simulink model "dedisp_sync"  (R2013b)
settings: Solver=FixedStepDiscrete  SolverMode=SingleTasking  StartTime=0.0  StopTime=10.0  RelTol=1e-3
undefined symbols (not defined in the file): pfb_coeff_gen_calc
libraries: xbsIndex_r4 x14646, casper_library_misc x70, casper_library_delays x55, dspsigops x16, xps_library x2, casper_library_pfbs x2
(part 19 of 146)

== system dedisp_sync/Parallel_Dedispersor_v11/Dedispersor_v2_1 ==
  Data : Inport
  Valid : Inport  Port=2
  Counter : xbsIndex_r4/Counter  cnt_type=Free Running  cnt_to=Inf  operation=Up  start_count=0  cnt_by_val=1  arith_type=Unsigned  n_bits=4  bin_pt=0  load_pin=off  rst=off  en=on  explicit_period=on  period=1  dbl_ovrd=off  use_behavioral_HDL=off  implementation=Fabric  block_type=counter
  Mux : xbsIndex_r4/Mux  inputs=16  en=off  latency=0  precision=Full  arith_type=Unsigned  n_bits=16  bin_pt=14  quantization=Truncate  overflow=Wrap  dbl_ovrd=off  block_type=mux
  detector_block_v2 : Subsystem  AncestorBlock=honestlibrary/detector_block_v2  mask(Basic block for FRB detection){chn=0, lat=1, nbits=4, behavioral=on}
      mask prompts: chn "Channel"; lat "Latency"; nbits "Number of Bits (Counter)"; behavioral "behavioral delay"
      mask help:
      | Delays a certain channel a number of latency clock cycles, according to the fixed DM table.
      | This version incorporates an internal counter (nbits) to know when store or give a certain value.
      mask init:
      | detector_block_init_v2(gcb,'chn',chn,'lat',lat,'nbits',nbits,'behavioral', behavioral)
      settings: AttributesFormatString=Channel: 0, Delay: 1
  detector_block_v21 : Subsystem  AncestorBlock=honestlibrary/detector_block_v2  mask(Basic block for FRB detection){chn=1, lat=2, nbits=4, behavioral=on}
      mask prompts: chn "Channel"; lat "Latency"; nbits "Number of Bits (Counter)"; behavioral "behavioral delay"
      mask help:
      | Delays a certain channel a number of latency clock cycles, according to the fixed DM table.
      | This version incorporates an internal counter (nbits) to know when store or give a certain value.
      mask init:
      | detector_block_init_v2(gcb,'chn',chn,'lat',lat,'nbits',nbits,'behavioral', behavioral)
      settings: AttributesFormatString=Channel: 1, Delay: 2
  detector_block_v210 : Subsystem  AncestorBlock=honestlibrary/detector_block_v2  mask(Basic block for FRB detection){chn=10, lat=11, nbits=4, behavioral=on}
      mask prompts: chn "Channel"; lat "Latency"; nbits "Number of Bits (Counter)"; behavioral "behavioral delay"
      mask help:
      | Delays a certain channel a number of latency clock cycles, according to the fixed DM table.
      | This version incorporates an internal counter (nbits) to know when store or give a certain value.
      mask init:
      | detector_block_init_v2(gcb,'chn',chn,'lat',lat,'nbits',nbits,'behavioral', behavioral)
      settings: AttributesFormatString=Channel: 10, Delay: 11
  detector_block_v211 : Subsystem  AncestorBlock=honestlibrary/detector_block_v2  mask(Basic block for FRB detection){chn=11, lat=12, nbits=4, behavioral=on}
      mask prompts: chn "Channel"; lat "Latency"; nbits "Number of Bits (Counter)"; behavioral "behavioral delay"
      mask help:
      | Delays a certain channel a number of latency clock cycles, according to the fixed DM table.
      | This version incorporates an internal counter (nbits) to know when store or give a certain value.
      mask init:
      | detector_block_init_v2(gcb,'chn',chn,'lat',lat,'nbits',nbits,'behavioral', behavioral)
      settings: AttributesFormatString=Channel: 11, Delay: 12
  detector_block_v212 : Subsystem  AncestorBlock=honestlibrary/detector_block_v2  mask(Basic block for FRB detection){chn=12, lat=13, nbits=4, behavioral=on}
      mask prompts: chn "Channel"; lat "Latency"; nbits "Number of Bits (Counter)"; behavioral "behavioral delay"
      mask help:
      | Delays a certain channel a number of latency clock cycles, according to the fixed DM table.
      | This version incorporates an internal counter (nbits) to know when store or give a certain value.
      mask init:
      | detector_block_init_v2(gcb,'chn',chn,'lat',lat,'nbits',nbits,'behavioral', behavioral)
      settings: AttributesFormatString=Channel: 12, Delay: 13
  detector_block_v213 : Subsystem  AncestorBlock=honestlibrary/detector_block_v2  mask(Basic block for FRB detection){chn=13, lat=14, nbits=4, behavioral=on}
      mask prompts: chn "Channel"; lat "Latency"; nbits "Number of Bits (Counter)"; behavioral "behavioral delay"
      mask help:
      | Delays a certain channel a number of latency clock cycles, according to the fixed DM table.
      | This version incorporates an internal counter (nbits) to know when store or give a certain value.
      mask init:
      | detector_block_init_v2(gcb,'chn',chn,'lat',lat,'nbits',nbits,'behavioral', behavioral)
      settings: AttributesFormatString=Channel: 13, Delay: 14
  detector_block_v214 : Subsystem  AncestorBlock=honestlibrary/detector_block_v2  mask(Basic block for FRB detection){chn=14, lat=15, nbits=4, behavioral=on}
      mask prompts: chn "Channel"; lat "Latency"; nbits "Number of Bits (Counter)"; behavioral "behavioral delay"
      mask help:
      | Delays a certain channel a number of latency clock cycles, according to the fixed DM table.
      | This version incorporates an internal counter (nbits) to know when store or give a certain value.
      mask init:
      | detector_block_init_v2(gcb,'chn',chn,'lat',lat,'nbits',nbits,'behavioral', behavioral)
      settings: AttributesFormatString=Channel: 14, Delay: 15
  detector_block_v215 : Subsystem  AncestorBlock=honestlibrary/detector_block_v2  mask(Basic block for FRB detection){chn=15, lat=16, nbits=4, behavioral=on}
      mask prompts: chn "Channel"; lat "Latency"; nbits "Number of Bits (Counter)"; behavioral "behavioral delay"
      mask help:
      | Delays a certain channel a number of latency clock cycles, according to the fixed DM table.
      | This version incorporates an internal counter (nbits) to know when store or give a certain value.
      mask init:
      | detector_block_init_v2(gcb,'chn',chn,'lat',lat,'nbits',nbits,'behavioral', behavioral)
      settings: AttributesFormatString=Channel: 15, Delay: 16
  detector_block_v22 : Subsystem  AncestorBlock=honestlibrary/detector_block_v2  mask(Basic block for FRB detection){chn=2, lat=3, nbits=4, behavioral=on}
      mask prompts: chn "Channel"; lat "Latency"; nbits "Number of Bits (Counter)"; behavioral "behavioral delay"
      mask help:
      | Delays a certain channel a number of latency clock cycles, according to the fixed DM table.
      | This version incorporates an internal counter (nbits) to know when store or give a certain value.
      mask init:
      | detector_block_init_v2(gcb,'chn',chn,'lat',lat,'nbits',nbits,'behavioral', behavioral)
      settings: AttributesFormatString=Channel: 2, Delay: 3
  detector_block_v23 : Subsystem  AncestorBlock=honestlibrary/detector_block_v2  mask(Basic block for FRB detection){chn=3, lat=4, nbits=4, behavioral=on}
      mask prompts: chn "Channel"; lat "Latency"; nbits "Number of Bits (Counter)"; behavioral "behavioral delay"
      mask help:
      | Delays a certain channel a number of latency clock cycles, according to the fixed DM table.
      | This version incorporates an internal counter (nbits) to know when store or give a certain value.
      mask init:
      | detector_block_init_v2(gcb,'chn',chn,'lat',lat,'nbits',nbits,'behavioral', behavioral)
      settings: AttributesFormatString=Channel: 3, Delay: 4
  detector_block_v24 : Subsystem  AncestorBlock=honestlibrary/detector_block_v2  mask(Basic block for FRB detection){chn=4, lat=5, nbits=4, behavioral=on}
      mask prompts: chn "Channel"; lat "Latency"; nbits "Number of Bits (Counter)"; behavioral "behavioral delay"
      mask help:
      | Delays a certain channel a number of latency clock cycles, according to the fixed DM table.
      | This version incorporates an internal counter (nbits) to know when store or give a certain value.
      mask init:
      | detector_block_init_v2(gcb,'chn',chn,'lat',lat,'nbits',nbits,'behavioral', behavioral)
      settings: AttributesFormatString=Channel: 4, Delay: 5
  detector_block_v25 : Subsystem  AncestorBlock=honestlibrary/detector_block_v2  mask(Basic block for FRB detection){chn=5, lat=6, nbits=4, behavioral=on}
      mask prompts: chn "Channel"; lat "Latency"; nbits "Number of Bits (Counter)"; behavioral "behavioral delay"
      mask help:
      | Delays a certain channel a number of latency clock cycles, according to the fixed DM table.
      | This version incorporates an internal counter (nbits) to know when store or give a certain value.
      mask init:
      | detector_block_init_v2(gcb,'chn',chn,'lat',lat,'nbits',nbits,'behavioral', behavioral)
      settings: AttributesFormatString=Channel: 5, Delay: 6
  detector_block_v26 : Subsystem  AncestorBlock=honestlibrary/detector_block_v2  mask(Basic block for FRB detection){chn=6, lat=7, nbits=4, behavioral=on}
      mask prompts: chn "Channel"; lat "Latency"; nbits "Number of Bits (Counter)"; behavioral "behavioral delay"
      mask help:
      | Delays a certain channel a number of latency clock cycles, according to the fixed DM table.
      | This version incorporates an internal counter (nbits) to know when store or give a certain value.
      mask init:
      | detector_block_init_v2(gcb,'chn',chn,'lat',lat,'nbits',nbits,'behavioral', behavioral)
      settings: AttributesFormatString=Channel: 6, Delay: 7
  detector_block_v27 : Subsystem  AncestorBlock=honestlibrary/detector_block_v2  mask(Basic block for FRB detection){chn=7, lat=8, nbits=4, behavioral=on}
      mask prompts: chn "Channel"; lat "Latency"; nbits "Number of Bits (Counter)"; behavioral "behavioral delay"
      mask help:
      | Delays a certain channel a number of latency clock cycles, according to the fixed DM table.
      | This version incorporates an internal counter (nbits) to know when store or give a certain value.
      mask init:
      | detector_block_init_v2(gcb,'chn',chn,'lat',lat,'nbits',nbits,'behavioral', behavioral)
      settings: AttributesFormatString=Channel: 7, Delay: 8
  detector_block_v28 : Subsystem  AncestorBlock=honestlibrary/detector_block_v2  mask(Basic block for FRB detection){chn=8, lat=9, nbits=4, behavioral=on}
      mask prompts: chn "Channel"; lat "Latency"; nbits "Number of Bits (Counter)"; behavioral "behavioral delay"
      mask help:
      | Delays a certain channel a number of latency clock cycles, according to the fixed DM table.
      | This version incorporates an internal counter (nbits) to know when store or give a certain value.
      mask init:
      | detector_block_init_v2(gcb,'chn',chn,'lat',lat,'nbits',nbits,'behavioral', behavioral)
      settings: AttributesFormatString=Channel: 8, Delay: 9
  detector_block_v29 : Subsystem  AncestorBlock=honestlibrary/detector_block_v2  mask(Basic block for FRB detection){chn=9, lat=10, nbits=4, behavioral=on}
      mask prompts: chn "Channel"; lat "Latency"; nbits "Number of Bits (Counter)"; behavioral "behavioral delay"
      mask help:
      | Delays a certain channel a number of latency clock cycles, according to the fixed DM table.
      | This version incorporates an internal counter (nbits) to know when store or give a certain value.
      mask init:
      | detector_block_init_v2(gcb,'chn',chn,'lat',lat,'nbits',nbits,'behavioral', behavioral)
      settings: AttributesFormatString=Channel: 9, Delay: 10
  Output : Outport
  wires:
  Mux/1 -> Output/1
  detector_block_v215/1(Out1) -> Mux/17
  detector_block_v214/1(Out1) -> Mux/16
  detector_block_v213/1(Out1) -> Mux/15
  detector_block_v212/1(Out1) -> Mux/14
  detector_block_v211/1(Out1) -> Mux/13
  detector_block_v210/1(Out1) -> Mux/12
  detector_block_v29/1(Out1) -> Mux/11
  detector_block_v28/1(Out1) -> Mux/10
  detector_block_v27/1(Out1) -> Mux/9
  detector_block_v26/1(Out1) -> Mux/8
  detector_block_v25/1(Out1) -> Mux/7
  detector_block_v24/1(Out1) -> Mux/6
  detector_block_v23/1(Out1) -> Mux/5
  detector_block_v22/1(Out1) -> Mux/4
  detector_block_v21/1(Out1) -> Mux/3
  detector_block_v2/1(Out1) -> Mux/2
  Counter/1 -> Mux/1
  Valid/1 -> Counter/1, detector_block_v215/2(Valid), detector_block_v214/2(Valid), detector_block_v213/2(Valid), detector_block_v212/2(Valid), detector_block_v211/2(Valid), detector_block_v210/2(Valid), detector_block_v29/2(Valid), detector_block_v28/2(Valid), detector_block_v27/2(Valid), detector_block_v26/2(Valid), detector_block_v25/2(Valid), detector_block_v24/2(Valid), detector_block_v23/2(Valid), detector_block_v22/2(Valid), detector_block_v21/2(Valid), detector_block_v2/2(Valid)
  Data/1 -> detector_block_v215/1(Data), detector_block_v214/1(Data), detector_block_v213/1(Data), detector_block_v212/1(Data), detector_block_v211/1(Data), detector_block_v210/1(Data), detector_block_v29/1(Data), detector_block_v28/1(Data), detector_block_v27/1(Data), detector_block_v26/1(Data), detector_block_v25/1(Data), detector_block_v24/1(Data), detector_block_v23/1(Data), detector_block_v22/1(Data), detector_block_v21/1(Data), detector_block_v2/1(Data)

== system dedisp_sync/Parallel_Dedispersor_v11/Dedispersor_v2_2 ==
  Data : Inport
  Valid : Inport  Port=2
  Counter : xbsIndex_r4/Counter  cnt_type=Free Running  cnt_to=Inf  operation=Up  start_count=0  cnt_by_val=1  arith_type=Unsigned  n_bits=4  bin_pt=0  load_pin=off  rst=off  en=on  explicit_period=on  period=1  dbl_ovrd=off  use_behavioral_HDL=off  implementation=Fabric  block_type=counter
  Mux : xbsIndex_r4/Mux  inputs=16  en=off  latency=0  precision=Full  arith_type=Unsigned  n_bits=16  bin_pt=14  quantization=Truncate  overflow=Wrap  dbl_ovrd=off  block_type=mux
  detector_block_v2 : Subsystem  AncestorBlock=honestlibrary/detector_block_v2  mask(Basic block for FRB detection){chn=0, lat=1, nbits=4, behavioral=on}
      mask prompts: chn "Channel"; lat "Latency"; nbits "Number of Bits (Counter)"; behavioral "behavioral delay"
      mask help:
      | Delays a certain channel a number of latency clock cycles, according to the fixed DM table.
      | This version incorporates an internal counter (nbits) to know when store or give a certain value.
      mask init:
      | detector_block_init_v2(gcb,'chn',chn,'lat',lat,'nbits',nbits,'behavioral', behavioral)
      settings: AttributesFormatString=Channel: 0, Delay: 1
  detector_block_v21 : Subsystem  AncestorBlock=honestlibrary/detector_block_v2  mask(Basic block for FRB detection){chn=1, lat=2, nbits=4, behavioral=on}
      mask prompts: chn "Channel"; lat "Latency"; nbits "Number of Bits (Counter)"; behavioral "behavioral delay"
      mask help:
      | Delays a certain channel a number of latency clock cycles, according to the fixed DM table.
      | This version incorporates an internal counter (nbits) to know when store or give a certain value.
      mask init:
      | detector_block_init_v2(gcb,'chn',chn,'lat',lat,'nbits',nbits,'behavioral', behavioral)
      settings: AttributesFormatString=Channel: 1, Delay: 2
  detector_block_v210 : Subsystem  AncestorBlock=honestlibrary/detector_block_v2  mask(Basic block for FRB detection){chn=10, lat=11, nbits=4, behavioral=on}
      mask prompts: chn "Channel"; lat "Latency"; nbits "Number of Bits (Counter)"; behavioral "behavioral delay"
      mask help:
      | Delays a certain channel a number of latency clock cycles, according to the fixed DM table.
      | This version incorporates an internal counter (nbits) to know when store or give a certain value.
      mask init:
      | detector_block_init_v2(gcb,'chn',chn,'lat',lat,'nbits',nbits,'behavioral', behavioral)
      settings: AttributesFormatString=Channel: 10, Delay: 11
  detector_block_v211 : Subsystem  AncestorBlock=honestlibrary/detector_block_v2  mask(Basic block for FRB detection){chn=11, lat=12, nbits=4, behavioral=on}
      mask prompts: chn "Channel"; lat "Latency"; nbits "Number of Bits (Counter)"; behavioral "behavioral delay"
      mask help:
      | Delays a certain channel a number of latency clock cycles, according to the fixed DM table.
      | This version incorporates an internal counter (nbits) to know when store or give a certain value.
      mask init:
      | detector_block_init_v2(gcb,'chn',chn,'lat',lat,'nbits',nbits,'behavioral', behavioral)
      settings: AttributesFormatString=Channel: 11, Delay: 12
  detector_block_v212 : Subsystem  AncestorBlock=honestlibrary/detector_block_v2  mask(Basic block for FRB detection){chn=12, lat=13, nbits=4, behavioral=on}
      mask prompts: chn "Channel"; lat "Latency"; nbits "Number of Bits (Counter)"; behavioral "behavioral delay"
      mask help:
      | Delays a certain channel a number of latency clock cycles, according to the fixed DM table.
      | This version incorporates an internal counter (nbits) to know when store or give a certain value.
      mask init:
      | detector_block_init_v2(gcb,'chn',chn,'lat',lat,'nbits',nbits,'behavioral', behavioral)
      settings: AttributesFormatString=Channel: 12, Delay: 13
  detector_block_v213 : Subsystem  AncestorBlock=honestlibrary/detector_block_v2  mask(Basic block for FRB detection){chn=13, lat=14, nbits=4, behavioral=on}
      mask prompts: chn "Channel"; lat "Latency"; nbits "Number of Bits (Counter)"; behavioral "behavioral delay"
      mask help:
      | Delays a certain channel a number of latency clock cycles, according to the fixed DM table.
      | This version incorporates an internal counter (nbits) to know when store or give a certain value.
      mask init:
      | detector_block_init_v2(gcb,'chn',chn,'lat',lat,'nbits',nbits,'behavioral', behavioral)
      settings: AttributesFormatString=Channel: 13, Delay: 14
  detector_block_v214 : Subsystem  AncestorBlock=honestlibrary/detector_block_v2  mask(Basic block for FRB detection){chn=14, lat=15, nbits=4, behavioral=on}
      mask prompts: chn "Channel"; lat "Latency"; nbits "Number of Bits (Counter)"; behavioral "behavioral delay"
      mask help:
      | Delays a certain channel a number of latency clock cycles, according to the fixed DM table.
      | This version incorporates an internal counter (nbits) to know when store or give a certain value.
      mask init:
      | detector_block_init_v2(gcb,'chn',chn,'lat',lat,'nbits',nbits,'behavioral', behavioral)
      settings: AttributesFormatString=Channel: 14, Delay: 15
  detector_block_v215 : Subsystem  AncestorBlock=honestlibrary/detector_block_v2  mask(Basic block for FRB detection){chn=15, lat=16, nbits=4, behavioral=on}
      mask prompts: chn "Channel"; lat "Latency"; nbits "Number of Bits (Counter)"; behavioral "behavioral delay"
      mask help:
      | Delays a certain channel a number of latency clock cycles, according to the fixed DM table.
      | This version incorporates an internal counter (nbits) to know when store or give a certain value.
      mask init:
      | detector_block_init_v2(gcb,'chn',chn,'lat',lat,'nbits',nbits,'behavioral', behavioral)
      settings: AttributesFormatString=Channel: 15, Delay: 16
  detector_block_v22 : Subsystem  AncestorBlock=honestlibrary/detector_block_v2  mask(Basic block for FRB detection){chn=2, lat=3, nbits=4, behavioral=on}
      mask prompts: chn "Channel"; lat "Latency"; nbits "Number of Bits (Counter)"; behavioral "behavioral delay"
      mask help:
      | Delays a certain channel a number of latency clock cycles, according to the fixed DM table.
      | This version incorporates an internal counter (nbits) to know when store or give a certain value.
      mask init:
      | detector_block_init_v2(gcb,'chn',chn,'lat',lat,'nbits',nbits,'behavioral', behavioral)
      settings: AttributesFormatString=Channel: 2, Delay: 3
  detector_block_v23 : Subsystem  AncestorBlock=honestlibrary/detector_block_v2  mask(Basic block for FRB detection){chn=3, lat=4, nbits=4, behavioral=on}
      mask prompts: chn "Channel"; lat "Latency"; nbits "Number of Bits (Counter)"; behavioral "behavioral delay"
      mask help:
      | Delays a certain channel a number of latency clock cycles, according to the fixed DM table.
      | This version incorporates an internal counter (nbits) to know when store or give a certain value.
      mask init:
      | detector_block_init_v2(gcb,'chn',chn,'lat',lat,'nbits',nbits,'behavioral', behavioral)
      settings: AttributesFormatString=Channel: 3, Delay: 4
  detector_block_v24 : Subsystem  AncestorBlock=honestlibrary/detector_block_v2  mask(Basic block for FRB detection){chn=4, lat=5, nbits=4, behavioral=on}
      mask prompts: chn "Channel"; lat "Latency"; nbits "Number of Bits (Counter)"; behavioral "behavioral delay"
      mask help:
      | Delays a certain channel a number of latency clock cycles, according to the fixed DM table.
      | This version incorporates an internal counter (nbits) to know when store or give a certain value.
      mask init:
      | detector_block_init_v2(gcb,'chn',chn,'lat',lat,'nbits',nbits,'behavioral', behavioral)
      settings: AttributesFormatString=Channel: 4, Delay: 5
  detector_block_v25 : Subsystem  AncestorBlock=honestlibrary/detector_block_v2  mask(Basic block for FRB detection){chn=5, lat=6, nbits=4, behavioral=on}
      mask prompts: chn "Channel"; lat "Latency"; nbits "Number of Bits (Counter)"; behavioral "behavioral delay"
      mask help:
      | Delays a certain channel a number of latency clock cycles, according to the fixed DM table.
      | This version incorporates an internal counter (nbits) to know when store or give a certain value.
      mask init:
      | detector_block_init_v2(gcb,'chn',chn,'lat',lat,'nbits',nbits,'behavioral', behavioral)
      settings: AttributesFormatString=Channel: 5, Delay: 6
  detector_block_v26 : Subsystem  AncestorBlock=honestlibrary/detector_block_v2  mask(Basic block for FRB detection){chn=6, lat=7, nbits=4, behavioral=on}
      mask prompts: chn "Channel"; lat "Latency"; nbits "Number of Bits (Counter)"; behavioral "behavioral delay"
      mask help:
      | Delays a certain channel a number of latency clock cycles, according to the fixed DM table.
      | This version incorporates an internal counter (nbits) to know when store or give a certain value.
      mask init:
      | detector_block_init_v2(gcb,'chn',chn,'lat',lat,'nbits',nbits,'behavioral', behavioral)
      settings: AttributesFormatString=Channel: 6, Delay: 7
  detector_block_v27 : Subsystem  AncestorBlock=honestlibrary/detector_block_v2  mask(Basic block for FRB detection){chn=7, lat=8, nbits=4, behavioral=on}
      mask prompts: chn "Channel"; lat "Latency"; nbits "Number of Bits (Counter)"; behavioral "behavioral delay"
      mask help:
      | Delays a certain channel a number of latency clock cycles, according to the fixed DM table.
      | This version incorporates an internal counter (nbits) to know when store or give a certain value.
      mask init:
      | detector_block_init_v2(gcb,'chn',chn,'lat',lat,'nbits',nbits,'behavioral', behavioral)
      settings: AttributesFormatString=Channel: 7, Delay: 8
  detector_block_v28 : Subsystem  AncestorBlock=honestlibrary/detector_block_v2  mask(Basic block for FRB detection){chn=8, lat=9, nbits=4, behavioral=on}
      mask prompts: chn "Channel"; lat "Latency"; nbits "Number of Bits (Counter)"; behavioral "behavioral delay"
      mask help:
      | Delays a certain channel a number of latency clock cycles, according to the fixed DM table.
      | This version incorporates an internal counter (nbits) to know when store or give a certain value.
      mask init:
      | detector_block_init_v2(gcb,'chn',chn,'lat',lat,'nbits',nbits,'behavioral', behavioral)
      settings: AttributesFormatString=Channel: 8, Delay: 9
  detector_block_v29 : Subsystem  AncestorBlock=honestlibrary/detector_block_v2  mask(Basic block for FRB detection){chn=9, lat=10, nbits=4, behavioral=on}
      mask prompts: chn "Channel"; lat "Latency"; nbits "Number of Bits (Counter)"; behavioral "behavioral delay"
      mask help:
      | Delays a certain channel a number of latency clock cycles, according to the fixed DM table.
      | This version incorporates an internal counter (nbits) to know when store or give a certain value.
      mask init:
      | detector_block_init_v2(gcb,'chn',chn,'lat',lat,'nbits',nbits,'behavioral', behavioral)
      settings: AttributesFormatString=Channel: 9, Delay: 10
  Output : Outport
  wires:
  Mux/1 -> Output/1
  detector_block_v215/1(Out1) -> Mux/17
  detector_block_v214/1(Out1) -> Mux/16
  detector_block_v213/1(Out1) -> Mux/15
  detector_block_v212/1(Out1) -> Mux/14
  detector_block_v211/1(Out1) -> Mux/13
  detector_block_v210/1(Out1) -> Mux/12
  detector_block_v29/1(Out1) -> Mux/11
  detector_block_v28/1(Out1) -> Mux/10
  detector_block_v27/1(Out1) -> Mux/9
  detector_block_v26/1(Out1) -> Mux/8
  detector_block_v25/1(Out1) -> Mux/7
  detector_block_v24/1(Out1) -> Mux/6
  detector_block_v23/1(Out1) -> Mux/5
  detector_block_v22/1(Out1) -> Mux/4
  detector_block_v21/1(Out1) -> Mux/3
  detector_block_v2/1(Out1) -> Mux/2
  Counter/1 -> Mux/1
  Valid/1 -> Counter/1, detector_block_v215/2(Valid), detector_block_v214/2(Valid), detector_block_v213/2(Valid), detector_block_v212/2(Valid), detector_block_v211/2(Valid), detector_block_v210/2(Valid), detector_block_v29/2(Valid), detector_block_v28/2(Valid), detector_block_v27/2(Valid), detector_block_v26/2(Valid), detector_block_v25/2(Valid), detector_block_v24/2(Valid), detector_block_v23/2(Valid), detector_block_v22/2(Valid), detector_block_v21/2(Valid), detector_block_v2/2(Valid)
  Data/1 -> detector_block_v215/1(Data), detector_block_v214/1(Data), detector_block_v213/1(Data), detector_block_v212/1(Data), detector_block_v211/1(Data), detector_block_v210/1(Data), detector_block_v29/1(Data), detector_block_v28/1(Data), detector_block_v27/1(Data), detector_block_v26/1(Data), detector_block_v25/1(Data), detector_block_v24/1(Data), detector_block_v23/1(Data), detector_block_v22/1(Data), detector_block_v21/1(Data), detector_block_v2/1(Data)

== system dedisp_sync/Parallel_Dedispersor_v11/Dedispersor_v2_3 ==
  Data : Inport
  Valid : Inport  Port=2
  Counter : xbsIndex_r4/Counter  cnt_type=Free Running  cnt_to=Inf  operation=Up  start_count=0  cnt_by_val=1  arith_type=Unsigned  n_bits=4  bin_pt=0  load_pin=off  rst=off  en=on  explicit_period=on  period=1  dbl_ovrd=off  use_behavioral_HDL=off  implementation=Fabric  block_type=counter
  Mux : xbsIndex_r4/Mux  inputs=16  en=off  latency=0  precision=Full  arith_type=Unsigned  n_bits=16  bin_pt=14  quantization=Truncate  overflow=Wrap  dbl_ovrd=off  block_type=mux
  detector_block_v2 : Subsystem  AncestorBlock=honestlibrary/detector_block_v2  mask(Basic block for FRB detection){chn=0, lat=1, nbits=4, behavioral=on}
      mask prompts: chn "Channel"; lat "Latency"; nbits "Number of Bits (Counter)"; behavioral "behavioral delay"
      mask help:
      | Delays a certain channel a number of latency clock cycles, according to the fixed DM table.
      | This version incorporates an internal counter (nbits) to know when store or give a certain value.
      mask init:
      | detector_block_init_v2(gcb,'chn',chn,'lat',lat,'nbits',nbits,'behavioral', behavioral)
      settings: AttributesFormatString=Channel: 0, Delay: 1
  detector_block_v21 : Subsystem  AncestorBlock=honestlibrary/detector_block_v2  mask(Basic block for FRB detection){chn=1, lat=2, nbits=4, behavioral=on}
      mask prompts: chn "Channel"; lat "Latency"; nbits "Number of Bits (Counter)"; behavioral "behavioral delay"
      mask help:
      | Delays a certain channel a number of latency clock cycles, according to the fixed DM table.
      | This version incorporates an internal counter (nbits) to know when store or give a certain value.
      mask init:
      | detector_block_init_v2(gcb,'chn',chn,'lat',lat,'nbits',nbits,'behavioral', behavioral)
      settings: AttributesFormatString=Channel: 1, Delay: 2
  detector_block_v210 : Subsystem  AncestorBlock=honestlibrary/detector_block_v2  mask(Basic block for FRB detection){chn=10, lat=11, nbits=4, behavioral=on}
      mask prompts: chn "Channel"; lat "Latency"; nbits "Number of Bits (Counter)"; behavioral "behavioral delay"
      mask help:
      | Delays a certain channel a number of latency clock cycles, according to the fixed DM table.
      | This version incorporates an internal counter (nbits) to know when store or give a certain value.
      mask init:
      | detector_block_init_v2(gcb,'chn',chn,'lat',lat,'nbits',nbits,'behavioral', behavioral)
      settings: AttributesFormatString=Channel: 10, Delay: 11
  detector_block_v211 : Subsystem  AncestorBlock=honestlibrary/detector_block_v2  mask(Basic block for FRB detection){chn=11, lat=12, nbits=4, behavioral=on}
      mask prompts: chn "Channel"; lat "Latency"; nbits "Number of Bits (Counter)"; behavioral "behavioral delay"
      mask help:
      | Delays a certain channel a number of latency clock cycles, according to the fixed DM table.
      | This version incorporates an internal counter (nbits) to know when store or give a certain value.
      mask init:
      | detector_block_init_v2(gcb,'chn',chn,'lat',lat,'nbits',nbits,'behavioral', behavioral)
      settings: AttributesFormatString=Channel: 11, Delay: 12
  detector_block_v212 : Subsystem  AncestorBlock=honestlibrary/detector_block_v2  mask(Basic block for FRB detection){chn=12, lat=13, nbits=4, behavioral=on}
      mask prompts: chn "Channel"; lat "Latency"; nbits "Number of Bits (Counter)"; behavioral "behavioral delay"
      mask help:
      | Delays a certain channel a number of latency clock cycles, according to the fixed DM table.
      | This version incorporates an internal counter (nbits) to know when store or give a certain value.
      mask init:
      | detector_block_init_v2(gcb,'chn',chn,'lat',lat,'nbits',nbits,'behavioral', behavioral)
      settings: AttributesFormatString=Channel: 12, Delay: 13
  detector_block_v213 : Subsystem  AncestorBlock=honestlibrary/detector_block_v2  mask(Basic block for FRB detection){chn=13, lat=14, nbits=4, behavioral=on}
      mask prompts: chn "Channel"; lat "Latency"; nbits "Number of Bits (Counter)"; behavioral "behavioral delay"
      mask help:
      | Delays a certain channel a number of latency clock cycles, according to the fixed DM table.
      | This version incorporates an internal counter (nbits) to know when store or give a certain value.
      mask init:
      | detector_block_init_v2(gcb,'chn',chn,'lat',lat,'nbits',nbits,'behavioral', behavioral)
      settings: AttributesFormatString=Channel: 13, Delay: 14
  detector_block_v214 : Subsystem  AncestorBlock=honestlibrary/detector_block_v2  mask(Basic block for FRB detection){chn=14, lat=15, nbits=4, behavioral=on}
      mask prompts: chn "Channel"; lat "Latency"; nbits "Number of Bits (Counter)"; behavioral "behavioral delay"
      mask help:
      | Delays a certain channel a number of latency clock cycles, according to the fixed DM table.
      | This version incorporates an internal counter (nbits) to know when store or give a certain value.
      mask init:
      | detector_block_init_v2(gcb,'chn',chn,'lat',lat,'nbits',nbits,'behavioral', behavioral)
      settings: AttributesFormatString=Channel: 14, Delay: 15
  detector_block_v215 : Subsystem  AncestorBlock=honestlibrary/detector_block_v2  mask(Basic block for FRB detection){chn=15, lat=16, nbits=4, behavioral=on}
      mask prompts: chn "Channel"; lat "Latency"; nbits "Number of Bits (Counter)"; behavioral "behavioral delay"
      mask help:
      | Delays a certain channel a number of latency clock cycles, according to the fixed DM table.
      | This version incorporates an internal counter (nbits) to know when store or give a certain value.
      mask init:
      | detector_block_init_v2(gcb,'chn',chn,'lat',lat,'nbits',nbits,'behavioral', behavioral)
      settings: AttributesFormatString=Channel: 15, Delay: 16
  detector_block_v22 : Subsystem  AncestorBlock=honestlibrary/detector_block_v2  mask(Basic block for FRB detection){chn=2, lat=3, nbits=4, behavioral=on}
      mask prompts: chn "Channel"; lat "Latency"; nbits "Number of Bits (Counter)"; behavioral "behavioral delay"
      mask help:
      | Delays a certain channel a number of latency clock cycles, according to the fixed DM table.
      | This version incorporates an internal counter (nbits) to know when store or give a certain value.
      mask init:
      | detector_block_init_v2(gcb,'chn',chn,'lat',lat,'nbits',nbits,'behavioral', behavioral)
      settings: AttributesFormatString=Channel: 2, Delay: 3
  detector_block_v23 : Subsystem  AncestorBlock=honestlibrary/detector_block_v2  mask(Basic block for FRB detection){chn=3, lat=4, nbits=4, behavioral=on}
      mask prompts: chn "Channel"; lat "Latency"; nbits "Number of Bits (Counter)"; behavioral "behavioral delay"
      mask help:
      | Delays a certain channel a number of latency clock cycles, according to the fixed DM table.
      | This version incorporates an internal counter (nbits) to know when store or give a certain value.
      mask init:
      | detector_block_init_v2(gcb,'chn',chn,'lat',lat,'nbits',nbits,'behavioral', behavioral)
      settings: AttributesFormatString=Channel: 3, Delay: 4
  detector_block_v24 : Subsystem  AncestorBlock=honestlibrary/detector_block_v2  mask(Basic block for FRB detection){chn=4, lat=5, nbits=4, behavioral=on}
      mask prompts: chn "Channel"; lat "Latency"; nbits "Number of Bits (Counter)"; behavioral "behavioral delay"
      mask help:
      | Delays a certain channel a number of latency clock cycles, according to the fixed DM table.
      | This version incorporates an internal counter (nbits) to know when store or give a certain value.
      mask init:
      | detector_block_init_v2(gcb,'chn',chn,'lat',lat,'nbits',nbits,'behavioral', behavioral)
      settings: AttributesFormatString=Channel: 4, Delay: 5
  detector_block_v25 : Subsystem  AncestorBlock=honestlibrary/detector_block_v2  mask(Basic block for FRB detection){chn=5, lat=6, nbits=4, behavioral=on}
      mask prompts: chn "Channel"; lat "Latency"; nbits "Number of Bits (Counter)"; behavioral "behavioral delay"
      mask help:
      | Delays a certain channel a number of latency clock cycles, according to the fixed DM table.
      | This version incorporates an internal counter (nbits) to know when store or give a certain value.
      mask init:
      | detector_block_init_v2(gcb,'chn',chn,'lat',lat,'nbits',nbits,'behavioral', behavioral)
      settings: AttributesFormatString=Channel: 5, Delay: 6
  detector_block_v26 : Subsystem  AncestorBlock=honestlibrary/detector_block_v2  mask(Basic block for FRB detection){chn=6, lat=7, nbits=4, behavioral=on}
      mask prompts: chn "Channel"; lat "Latency"; nbits "Number of Bits (Counter)"; behavioral "behavioral delay"
      mask help:
      | Delays a certain channel a number of latency clock cycles, according to the fixed DM table.
      | This version incorporates an internal counter (nbits) to know when store or give a certain value.
      mask init:
      | detector_block_init_v2(gcb,'chn',chn,'lat',lat,'nbits',nbits,'behavioral', behavioral)
      settings: AttributesFormatString=Channel: 6, Delay: 7
  detector_block_v27 : Subsystem  AncestorBlock=honestlibrary/detector_block_v2  mask(Basic block for FRB detection){chn=7, lat=8, nbits=4, behavioral=on}
      mask prompts: chn "Channel"; lat "Latency"; nbits "Number of Bits (Counter)"; behavioral "behavioral delay"
      mask help:
      | Delays a certain channel a number of latency clock cycles, according to the fixed DM table.
      | This version incorporates an internal counter (nbits) to know when store or give a certain value.
      mask init:
      | detector_block_init_v2(gcb,'chn',chn,'lat',lat,'nbits',nbits,'behavioral', behavioral)
      settings: AttributesFormatString=Channel: 7, Delay: 8
  detector_block_v28 : Subsystem  AncestorBlock=honestlibrary/detector_block_v2  mask(Basic block for FRB detection){chn=8, lat=9, nbits=4, behavioral=on}
      mask prompts: chn "Channel"; lat "Latency"; nbits "Number of Bits (Counter)"; behavioral "behavioral delay"
      mask help:
      | Delays a certain channel a number of latency clock cycles, according to the fixed DM table.
      | This version incorporates an internal counter (nbits) to know when store or give a certain value.
      mask init:
      | detector_block_init_v2(gcb,'chn',chn,'lat',lat,'nbits',nbits,'behavioral', behavioral)
      settings: AttributesFormatString=Channel: 8, Delay: 9
  detector_block_v29 : Subsystem  AncestorBlock=honestlibrary/detector_block_v2  mask(Basic block for FRB detection){chn=9, lat=10, nbits=4, behavioral=on}
      mask prompts: chn "Channel"; lat "Latency"; nbits "Number of Bits (Counter)"; behavioral "behavioral delay"
      mask help:
      | Delays a certain channel a number of latency clock cycles, according to the fixed DM table.
      | This version incorporates an internal counter (nbits) to know when store or give a certain value.
      mask init:
      | detector_block_init_v2(gcb,'chn',chn,'lat',lat,'nbits',nbits,'behavioral', behavioral)
      settings: AttributesFormatString=Channel: 9, Delay: 10
  Output : Outport
  wires:
  Mux/1 -> Output/1
  detector_block_v215/1(Out1) -> Mux/17
  detector_block_v214/1(Out1) -> Mux/16
  detector_block_v213/1(Out1) -> Mux/15
  detector_block_v212/1(Out1) -> Mux/14
  detector_block_v211/1(Out1) -> Mux/13
  detector_block_v210/1(Out1) -> Mux/12
  detector_block_v29/1(Out1) -> Mux/11
  detector_block_v28/1(Out1) -> Mux/10
  detector_block_v27/1(Out1) -> Mux/9
  detector_block_v26/1(Out1) -> Mux/8
  detector_block_v25/1(Out1) -> Mux/7
  detector_block_v24/1(Out1) -> Mux/6
  detector_block_v23/1(Out1) -> Mux/5
  detector_block_v22/1(Out1) -> Mux/4
  detector_block_v21/1(Out1) -> Mux/3
  detector_block_v2/1(Out1) -> Mux/2
  Counter/1 -> Mux/1
  Valid/1 -> Counter/1, detector_block_v215/2(Valid), detector_block_v214/2(Valid), detector_block_v213/2(Valid), detector_block_v212/2(Valid), detector_block_v211/2(Valid), detector_block_v210/2(Valid), detector_block_v29/2(Valid), detector_block_v28/2(Valid), detector_block_v27/2(Valid), detector_block_v26/2(Valid), detector_block_v25/2(Valid), detector_block_v24/2(Valid), detector_block_v23/2(Valid), detector_block_v22/2(Valid), detector_block_v21/2(Valid), detector_block_v2/2(Valid)
  Data/1 -> detector_block_v215/1(Data), detector_block_v214/1(Data), detector_block_v213/1(Data), detector_block_v212/1(Data), detector_block_v211/1(Data), detector_block_v210/1(Data), detector_block_v29/1(Data), detector_block_v28/1(Data), detector_block_v27/1(Data), detector_block_v26/1(Data), detector_block_v25/1(Data), detector_block_v24/1(Data), detector_block_v23/1(Data), detector_block_v22/1(Data), detector_block_v21/1(Data), detector_block_v2/1(Data)
